simulink model "linear"  (Simulink 6.1)
settings: Solver=ode45  SolverMode=SingleTasking  StartTime=Tmin  StopTime=Tmax  FixedStep=0.001  RelTol=1e-3
values from neighbouring files (symbols this model uses):
  height = 3    [truckresponse.m]
  k = 3500    [truckresponse.m]
  m = 150    [truckresponse.m]
undefined symbols (not defined in the file or in its folder): b
settings Model: LastModifiedBy=m134506  ExtModeArmWhenConnect=off  BufferReuse=off
settings DataIOCC: LimitDataPoints=off  TimeSaveName=tlin  Refine=100
settings OptimizationCC: BooleanDataType=off  OptimizeBlockIOStorage=off  BufferReuse=off  ExpressionFolding=off  LocalBlockOutputs=off
settings DebuggingCC: SolverPrmCheckMsg=warning
settings RTWCC: SystemTargetFile=wincon.tlc  MakeCommand=make_wc  TemplateMakefile=wc_default_tmf  Description=WinCon Target  ProcessScript=wincon_make_rtw_hook
settings STFCustomTargetCC: TargetFcnLib=ansi_tfl_tmw.mat  GenFloatMathFcnCalls=ANSI_C  ModelReferenceCompliant=off  SystemTargetFile=wincon.tlc
settings GRTTargetCC: ModelReferenceCompliant=off  MatFileLogging=off  ExtMode=on  ExtModeTransport=2  ExtModeMexFile=wc_comm
settings CustomProperty: Value=on

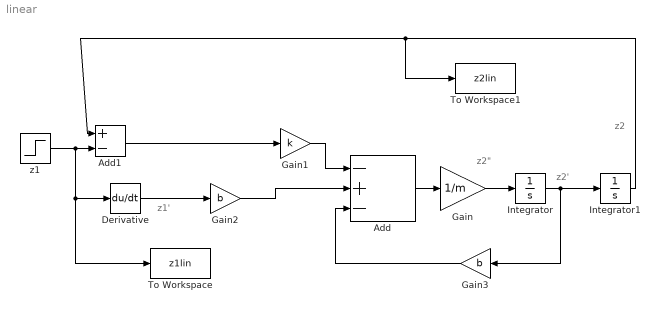
== system linear ==
  note: z2"
  note: z2'
  note: z2
  note: z1'
  Add : Sum  Inputs=-+-  OutScaling=2^-10
  Add1 : Sum  Inputs=+-  OutScaling=2^-10
  Derivative : Derivative
  Gain : Gain  Gain=1/m
  Gain1 : Gain  Gain=k
  Gain2 : Gain  Gain=b
  Gain3 : Gain  Orientation=left  Gain=b
  Integrator : Integrator
  Integrator1 : Integrator
  To Workspace : ToWorkspace  VariableName=z1lin  SampleTime=-1  SaveFormat=Array
  To Workspace1 : ToWorkspace  VariableName=z2lin  SampleTime=-1  SaveFormat=Array
  z1 : Step  Time=0  After=height  SampleTime=0
  wires:
  z1/1 -> Add1/2, Derivative/1, To Workspace/1
  Add/1 -> Gain/1
  Gain/1 -> Integrator/1
  Integrator/1 -> Integrator1/1, Gain3/1
  Derivative/1 -> Gain2/1
  Integrator1/1 -> Add1/1, To Workspace1/1
  Gain1/1 -> Add/1
  Gain2/1 -> Add/2
  Gain3/1 -> Add/3
  Add1/1 -> Gain1/1
